simulink model "Dclab_Session6"  (R2018b)
settings: Solver=VariableStepAuto  StartTime=0.0  StopTime=0.5  RelTol=1e-3
InitFcn:
  | run('TxEncoder.m')
values from neighbouring files (symbols this model uses):
  alpha = 0.2    [TxEncoder.m]
  filter_coeff = fliplr(Header(2:end).*conj(Header(1:end-1)))    [TxEncoder.m]
  N_Frame = 3*N_data + 2*N_pilot + N_header    (= 943)    [TxEncoder.m]
  Rs = 1e6    (= 1000000)    [TxEncoder.m]
  Sps = 8    [TxEncoder.m]
undefined symbols (not defined in the file or in its folder): Frame, magnitude
libraries: commdigbbndpm3 x5, simulink x3, commfilt2 x2, commchan3 x1, dspstat3 x1
settings Model: Creator=DATiS  LastModifiedBy=amira
settings DataIOCC: ReturnWorkspaceOutputs=on

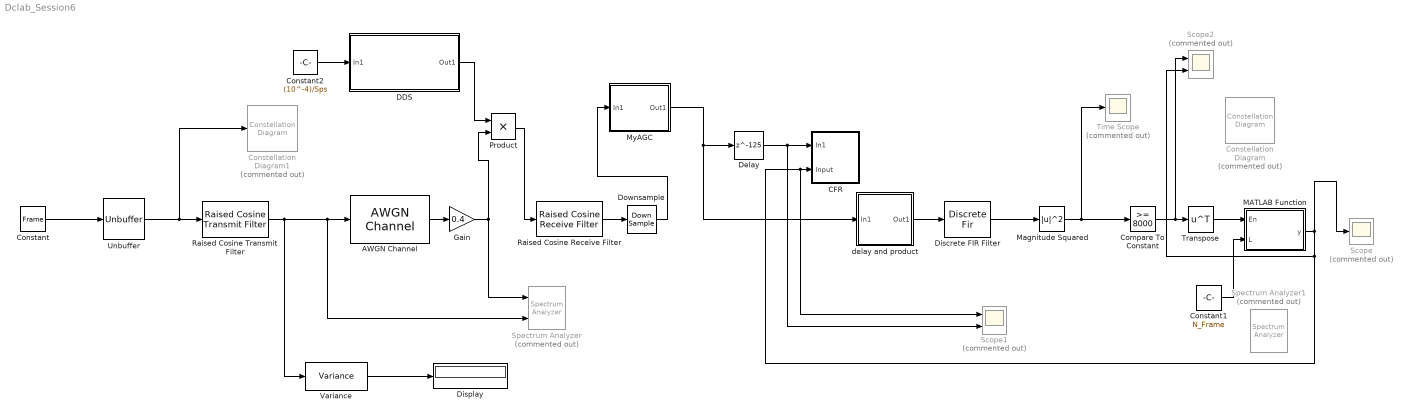
== system Dclab_Session6 ==
  AWGN Channel : commchan3/AWGN Channel  InputProcessing=Columns as channels (frame based)  seed=67  noiseMode="Signal to noise ratio  (Es/No)"  EbNodB=10  EsNodB=ESN0  SNRdB=10  bitsPerSym=1  Ps=1/Sps  Tsym=1/Rs  variance=1
      settings: SourceProductName=Communications Toolbox
  "CFR " : Subsystem
  Compare To Constant : simulink/Logic and Bit Operations/Compare To Constant  relop=>=  const=8000  OutDataTypeStr=boolean
  Constant : Constant  Value=Frame  SampleTime=length(Frame)/Rs
  Constant1 : Constant  Value=N_Frame  SampleTime=1/Rs
  Constant2 : Constant  Value=(10^-4)/Sps
  Constellation Diagram : ConstellationDiagram  Commented=on
  Constellation Diagram1 : ConstellationDiagram  Commented=on
  DDS : Subsystem
  Delay : Delay  DelayLength=125
  Discrete FIR Filter : DiscreteFir  Coefficients=filter_coeff
  Display : Display
  Downsample : DownSample  N=Sps  RateOptions=Allow multirate processing
  Gain : Gain  Gain=0.4
  MATLAB Function : MATLAB Function  TreatAsAtomicUnit=on
  Magnitude Squared : Math  Operator=magnitude^2  SaturateOnIntegerOverflow=on
  "MyAGC " : Subsystem
  Product : Product
  Raised Cosine Receive Filter : commfilt2/Raised Cosine Receive Filter  filtType=Square root  R=alpha  filtSpan=Span  N=Sps  downFactor=1  downOffset=0  filterGain=1  RateOptions=Allow multirate processing  framing=Mute  checkCoeff=off  variableName=rcRxFilt  currentFiltSpan=20  D=(20)/2  inputOffset=0  sampMode=Mute  saveAsFlag=0  rateMode=Downsampling  checkGain=Normalized  launchFVT=on  roundingMode=Floor  overflowMode=off  coeffDataTypeStr=Inherit: Same word length as input  coeffMin=[]  coeffMax=[]  coeffLastDataTypeStr=Inherit: Same word length as input  accumDataTypeStr=Inherit: Same as product output  accumLastDataTypeStr=Inherit: Same as product output  outputDataTypeStr=Inherit: Same as accumulator  outputMin=[]  outputMax=[]  outputLastDataTypeStr=Inherit: Same as accumulator
      settings: SourceProductName=Communications Toolbox
  Raised Cosine Transmit Filter : commfilt2/Raised Cosine Transmit Filter  filtType=Square root  R=alpha  filtSpan=Span  N=Sps  filterGain=1  RateOptions=Allow multirate processing  framing=Mute  checkCoeff=off  variableName=rcTxFilt  checkGain=Normalized  sampMode=Mute  saveAsFlag=0  currentFiltSpan=20  D=(20)/2  launchFVT=on  roundingMode=Floor  overflowMode=off  coeffDataTypeStr=Inherit: Same word length as input  coeffMin=[]  coeffMax=[]  coeffLastDataTypeStr=Inherit: Same word length as input  outputDataTypeStr=Inherit: Same as accumulator  outputMin=[]  outputMax=[]  outputLastDataTypeStr=Inherit: Same as accumulator
      settings: SourceProductName=Communications Toolbox
  Scope : Scope  Commented=on
  Scope1 : Scope  Commented=on  NumInputPorts=2
  Scope2 : Scope  Commented=on  NumInputPorts=2
  Spectrum Analyzer : SpectrumAnalyzer  Commented=on  NumInputPorts=2
  Spectrum Analyzer1 : SpectrumAnalyzer  Commented=on
  Time Scope : Scope  Commented=on
  Transpose : Math  Operator=transpose  SaturateOnIntegerOverflow=on
  Unbuffer : Unbuffer
  Variance : dspstat3/Variance  run=on  reset_popup=None  directionMode=Each column  dimension=1  roiEnable=off  roiType=Rectangles  roiPortion=Entire ROI  roiOutput=Individual statistics for each ROI  roiFlag=off  roundingMode=Floor  overflowMode=off
      settings: SourceProductName=DSP System Toolbox
  delay and product : Subsystem
  wires:
  AWGN Channel/1 -> Gain/1
  Raised Cosine Receive Filter/1 -> Downsample/1
  Variance/1 -> Display/1
  Constant/1 -> Unbuffer/1
  Unbuffer/1 -> Constellation Diagram1/1, Raised Cosine Transmit Filter/1
  Discrete FIR Filter/1 -> Magnitude Squared/1
  Magnitude Squared/1 -> Time Scope/1, Compare To Constant/1
  delay and product/1(Out1) -> Discrete FIR Filter/1
  Constant1/1 -> MATLAB Function/2(L)
  Compare To Constant/1 -> Scope2/1, Transpose/1
  Transpose/1 -> MATLAB Function/1(En)
  Downsample/1 -> "MyAGC "/1(In1)
  Raised Cosine Transmit Filter/1 -> Variance/1, AWGN Channel/1, Spectrum Analyzer/2
  MATLAB Function/1(y) -> Scope2/2, Scope1/1, "CFR "/2(Input), Scope/1
  Delay/1 -> Scope1/2, "CFR "/1(In1)
  "MyAGC "/1(Out1) -> delay and product/1(In1), Delay/1
  Gain/1 -> Spectrum Analyzer/1, Product/2
  Product/1 -> Raised Cosine Receive Filter/1
  Constant2/1 -> DDS/1(In1)
  DDS/1(Out1) -> Product/1

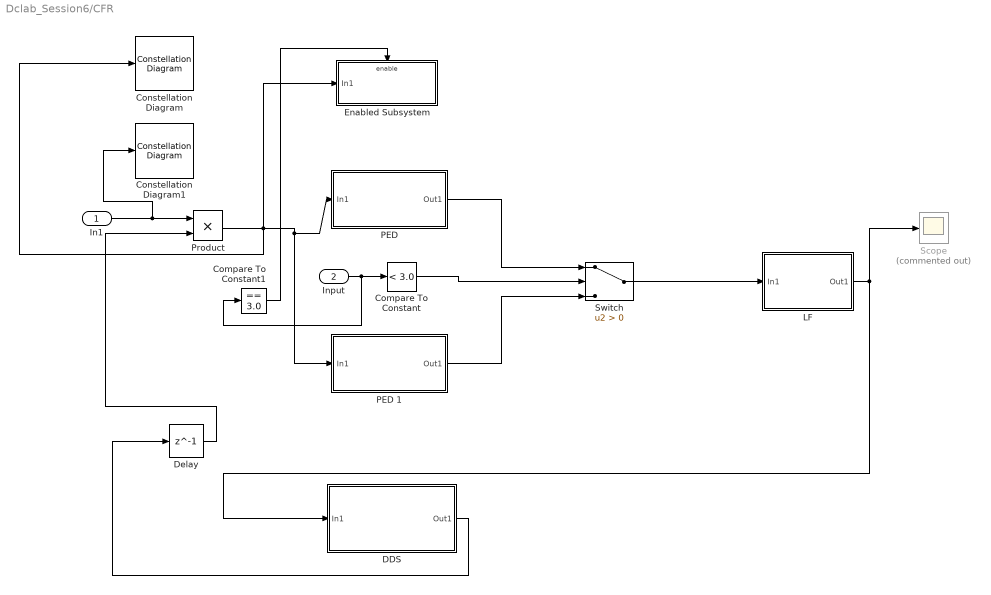
== system Dclab_Session6/CFR  ==
  In1 : Inport
  Input : Inport  Port=2
  Compare To Constant : simulink/Logic and Bit Operations/Compare To Constant  relop=<  const=3.0  OutDataTypeStr=boolean
  Compare To Constant1 : simulink/Logic and Bit Operations/Compare To Constant  relop===  const=3.0  OutDataTypeStr=boolean
  Constellation Diagram : ConstellationDiagram
  Constellation Diagram1 : ConstellationDiagram
  DDS : Subsystem
  Delay : Delay  DelayLength=1
  Enabled Subsystem : Subsystem  TreatAsAtomicUnit=on
  "LF " : Subsystem
  "PED " : Subsystem
  PED 1 : Subsystem
  Product : Product
  Scope : Scope  Commented=on
  Switch : Switch  Criteria=u2 > Threshold
  wires:
  "LF "/1(Out1) -> Scope/1, DDS/1(In1)
  In1/1 -> Constellation Diagram1/1, Product/1
  DDS/1(Out1) -> Delay/1
  Delay/1 -> Product/2
  Product/1 -> Enabled Subsystem/1(In1), Constellation Diagram/1, PED 1/1(In1), "PED "/1(In1)
  "PED "/1(Out1) -> Switch/1
  PED 1/1(Out1) -> Switch/3
  Compare To Constant/1 -> Switch/2
  Input/1 -> Compare To Constant1/1, Compare To Constant/1
  Switch/1 -> "LF "/1(In1)
  Compare To Constant1/1 -> Enabled Subsystem/Enable

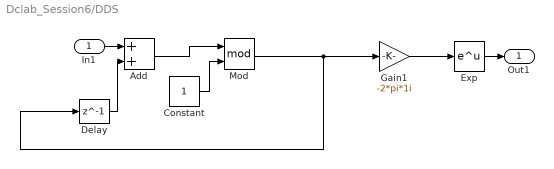
== system Dclab_Session6/DDS ==
  In1 : Inport
  Add : Sum
  Constant : Constant  SampleTime=1/Rs
  Delay : Delay  DelayLength=1
  Exp : Math  SaturateOnIntegerOverflow=on
  Gain1 : Gain  Gain=-2*pi*1i
  Mod : Math  Operator=mod  SaturateOnIntegerOverflow=on
  Out1 : Outport
  wires:
  Mod/1 -> Delay/1, Gain1/1
  Gain1/1 -> Exp/1
  Delay/1 -> Add/2
  In1/1 -> Add/1
  Exp/1 -> Out1/1
  Add/1 -> Mod/1
  Constant/1 -> Mod/2

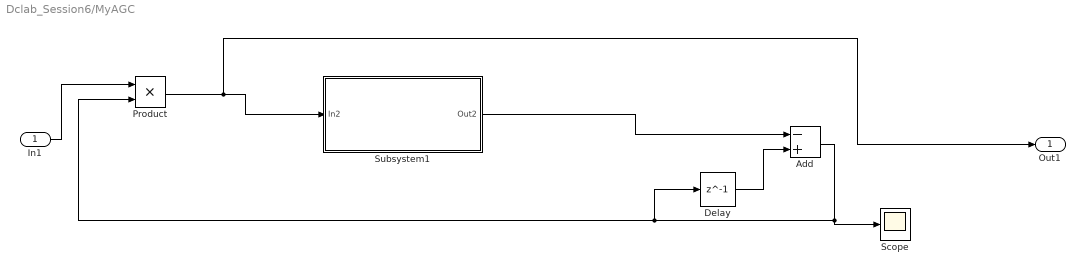
== system Dclab_Session6/MyAGC  ==
  In1 : Inport
  Add : Sum  Inputs=-+
  Delay : Delay  DelayLength=1  InitialCondition=1
  Product : Product
  Scope : Scope
  Subsystem1 : Subsystem
  Out1 : Outport
  wires:
  Delay/1 -> Add/2
  Add/1 -> Scope/1, Product/2, Delay/1
  Subsystem1/1(Out2) -> Add/1
  In1/1 -> Product/1
  Product/1 -> Out1/1, Subsystem1/1(In2)

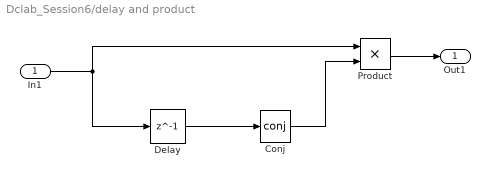
== system Dclab_Session6/delay and product ==
  In1 : Inport
  Conj : Math  Operator=conj  SaturateOnIntegerOverflow=on
  Delay : Delay  DelayLength=1
  Product : Product
  Out1 : Outport  VectorParamsAs1DForOutWhenUnconnected=on
  wires:
  Conj/1 -> Product/2
  Product/1 -> Out1/1
  In1/1 -> Product/1, Delay/1
  Delay/1 -> Conj/1

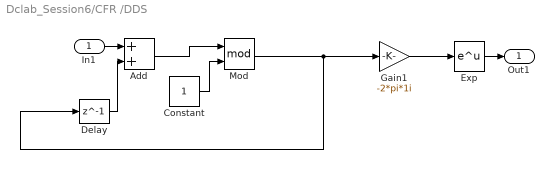
== system Dclab_Session6/CFR /DDS ==
  In1 : Inport
  Add : Sum
  Constant : Constant  SampleTime=1/Rs
  Delay : Delay  DelayLength=1
  Exp : Math  SaturateOnIntegerOverflow=on
  Gain1 : Gain  Gain=-2*pi*1i
  Mod : Math  Operator=mod  SaturateOnIntegerOverflow=on
  Out1 : Outport
  wires:
  Mod/1 -> Delay/1, Gain1/1
  Gain1/1 -> Exp/1
  Delay/1 -> Add/2
  In1/1 -> Add/1
  Exp/1 -> Out1/1
  Add/1 -> Mod/1
  Constant/1 -> Mod/2

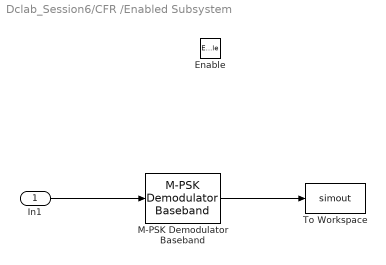
== system Dclab_Session6/CFR /Enabled Subsystem ==
  In1 : Inport
  Enable : EnablePort
  M-PSK Demodulator Baseband : commdigbbndpm3/M-PSK Demodulator Baseband  M=8  OutType=Integer  DecType=Hard decision  VarSource=Dialog  Variance=1  Dec=Gray  Mapping=[0:7]  Ph=pi/8  outDtype1=Inherit via internal rule  outDtype2=Inherit via internal rule  derotateFactorWordLen=16  derotateFactorDataTypeStr=Inherit: Same word length as input  derotateFactorLastDataTypeStr=Inherit: Same word length as input
      settings: SourceProductName=Communications System Toolbox
  To Workspace : ToWorkspace  VariableName=simout  SampleTime=-1
      settings: Save2DSignal=2-D array (concatenate along first dimension)
  wires:
  In1/1 -> M-PSK Demodulator Baseband/1
  M-PSK Demodulator Baseband/1 -> To Workspace/1

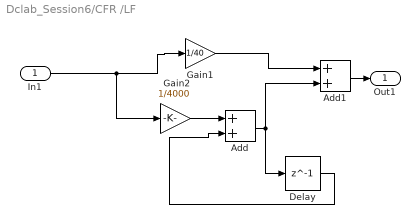
== system Dclab_Session6/CFR /LF  ==
  In1 : Inport
  Add : Sum
  Add1 : Sum
  Delay : Delay  DelayLength=1
  Gain1 : Gain  Gain=1/40
  Gain2 : Gain  Gain=1/4000
  Out1 : Outport
  wires:
  Delay/1 -> Add/2
  Add1/1 -> Out1/1
  Gain2/1 -> Add/1
  Add/1 -> Add1/2, Delay/1
  Gain1/1 -> Add1/1
  In1/1 -> Gain2/1, Gain1/1

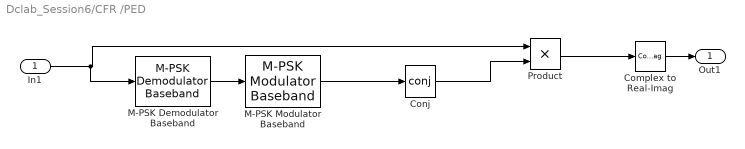
== system Dclab_Session6/CFR /PED  ==
  In1 : Inport
  Complex to Real-Imag : ComplexToRealImag  Output=Imag
  Conj : Math  Operator=conj  SaturateOnIntegerOverflow=on
  M-PSK Demodulator Baseband : commdigbbndpm3/M-PSK Demodulator Baseband  M=2  OutType=Integer  DecType=Hard decision  VarSource=Dialog  Variance=1  Dec=Gray  Mapping=[0:7]  Ph=0  outDtype1=Inherit via internal rule  outDtype2=Inherit via internal rule  derotateFactorWordLen=16  derotateFactorDataTypeStr=Inherit: Same word length as input  derotateFactorLastDataTypeStr=Inherit: Same word length as input
      settings: SourceProductName=Communications System Toolbox
  M-PSK Modulator Baseband : commdigbbndpm3/M-PSK Modulator Baseband  M=2  InType=Integer  Enc=Gray  Mapping=[0:7]  Ph=0  outDtype=double  outWordLen=16  outUDDataType=sfix(16)  outFracLenMode=Best precision  outFracLen=15  outDataTypeStr=double  outLastDataTypeStr=double
      settings: SourceProductName=Communications System Toolbox
  Product : Product
  Out1 : Outport
  wires:
  M-PSK Demodulator Baseband/1 -> M-PSK Modulator Baseband/1
  M-PSK Modulator Baseband/1 -> Conj/1
  Conj/1 -> Product/2
  Product/1 -> Complex to Real-Imag/1
  In1/1 -> M-PSK Demodulator Baseband/1, Product/1
  Complex to Real-Imag/1 -> Out1/1

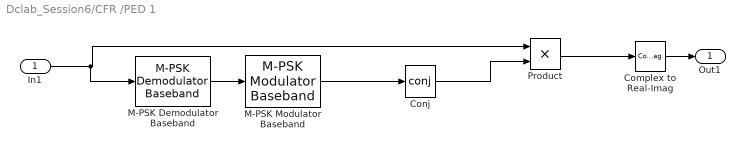
== system Dclab_Session6/CFR /PED 1 ==
  In1 : Inport
  Complex to Real-Imag : ComplexToRealImag  Output=Imag
  Conj : Math  Operator=conj  SaturateOnIntegerOverflow=on
  M-PSK Demodulator Baseband : commdigbbndpm3/M-PSK Demodulator Baseband  M=Mode_order  OutType=Integer  DecType=Hard decision  VarSource=Dialog  Variance=1  Dec=Gray  Mapping=[0:7]  Ph=Phase_offset  outDtype1=Inherit via internal rule  outDtype2=Inherit via internal rule  derotateFactorWordLen=16  derotateFactorDataTypeStr=Inherit: Same word length as input  derotateFactorLastDataTypeStr=Inherit: Same word length as input
      settings: SourceProductName=Communications System Toolbox
  M-PSK Modulator Baseband : commdigbbndpm3/M-PSK Modulator Baseband  M=Mode_order  InType=Integer  Enc=Gray  Mapping=[0:7]  Ph=Phase_offset  outDtype=double  outWordLen=16  outUDDataType=sfix(16)  outFracLenMode=Best precision  outFracLen=15  outDataTypeStr=double  outLastDataTypeStr=double
      settings: SourceProductName=Communications System Toolbox
  Product : Product
  Out1 : Outport
  wires:
  M-PSK Demodulator Baseband/1 -> M-PSK Modulator Baseband/1
  M-PSK Modulator Baseband/1 -> Conj/1
  Conj/1 -> Product/2
  Product/1 -> Complex to Real-Imag/1
  In1/1 -> M-PSK Demodulator Baseband/1, Product/1
  Complex to Real-Imag/1 -> Out1/1

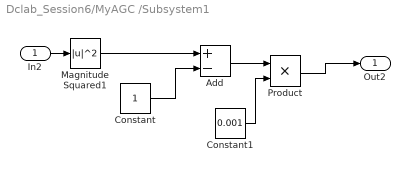
== system Dclab_Session6/MyAGC /Subsystem1 ==
  In2 : Inport
  Add : Sum  Inputs=+-
  Constant : Constant
  Constant1 : Constant  Value=0.001
  Magnitude Squared1 : Math  Operator=magnitude^2  SaturateOnIntegerOverflow=on
  Product : Product
  Out2 : Outport
  wires:
  Constant/1 -> Add/2
  Magnitude Squared1/1 -> Add/1
  In2/1 -> Magnitude Squared1/1
  Add/1 -> Product/1
  Constant1/1 -> Product/2
  Product/1 -> Out2/1

== matlab function Dclab_Session6/MATLAB Function ==
  data: En input; y output; L input
function y = fcn(En, L)
persistent count
if isempty(count)
   count = 0; 
end

if (En(1))
   count = 0; 
end

count = mod(count + 1, L);
y = 0;
if count <= 126
    y = 1;
elseif count <= 126+256
    y = 3;
elseif count <= 126+256+24
    y = 2;
elseif count <= 126+256+24+256
    y = 3;
elseif count <= 126+256+24+256+24
    y = 2;
else
    y = 3; 
end

end
